simulink model "AHRS_voter_Harness3"  (R2018b)
settings: Solver=FixedStepDiscrete  StartTime=0.0  StopTime=10.0  FixedStep=0.01  RelTol=1e-3  EnableMultiTasking=on
Description:
  | Harness for testing 3 valid AHRS
settings Model: Creator=bpotter  LastModifiedBy=bpotter
settings DataIOCC: LimitDataPoints=on  SaveOutput=off  DSMLogging=off  InspectSignalLogs=on  SaveTime=off
settings OptimizationCC: BlockReduction=off  DefaultParameterBehavior=Inlined  InitFltsAndDblsToZero=on  EfficientFloat2IntCast=on  EfficientMapNaN2IntZero=off  LifeSpan=inf  MaxStackSize=inf
settings DebuggingCC: SignalInfNanChecking=error  SignalRangeChecking=error  ReadBeforeWriteMsg=EnableAllAsError  WriteAfterWriteMsg=EnableAllAsError  WriteAfterReadMsg=EnableAllAsError  AlgebraicLoopMsg=error  ArtificialAlgebraicLoopMsg=error  SaveWithDisabledLinksMsg=error  SaveWithParameterizedLinksMsg=error  BlockPriorityViolationMsg=error  SolverPrmCheckMsg=error  InheritedTsInSrcMsg=error  SigSpecEnsureSampleTimeMsg=error  CheckMatrixSingularityMsg=error  IntegerOverflowMsg=error  ParameterUnderflowMsg=error  ParameterPrecisionLossMsg=error  ParameterTunabilityLossMsg=error  UnderSpecifiedDataTypeMsg=error  UnnecessaryDatatypeConvMsg=warning  VectorMatrixConversionMsg=error  SignalLabelMismatchMsg=error  UnconnectedInputMsg=error  UnconnectedOutputMsg=error  UnconnectedLineMsg=error  SFcnCompatibilityMsg=error  BusObjectLabelMismatch=error  RootOutportRequireBusObject=error  AssertControl=DisableAll  AllowSymbolicDim=off  ModelReferenceIOMsg=error  ModelReferenceIOMismatchMessage=error  UnknownTsInhSupMsg=error  ModelReferenceDataLoggingMessage=error  StateNameClashWarn=warning  StrictBusMsg=ErrorOnBusTreatedAsVector  NonBusSignalsTreatedAsBus=error  SFInvalidInputDataAccessInChartInitDiag=error  SFTransitionOutsideNaturalParentDiag=error  SFUnreachableExecutionPathDiag=error  SFUndirectedBroadcastEventsDiag=error  SFTransitionActionBeforeConditionDiag=error  IntegerSaturationMsg=error
settings HardwareCC: ProdBitPerPointer=32  ProdBitPerSizeT=32  ProdBitPerPtrDiffT=32  ProdLargestAtomicFloat=None  ProdEndianess=Unspecified  ProdWordSize=32  ProdHWDeviceType=32-bit Generic  TargetIntDivRoundTo=Zero
settings ModelReferenceCC: PropagateSignalLabelsOutOfModel=off
settings SFSimCC: SimUseLocalCustomCode=off  MATLABDynamicMemAlloc=off
settings RTWCC: SystemTargetFile=ert.tlc  TemplateMakefile=ert_default_tmf  GenerateReport=on  RTWUseLocalCustomCode=off  IncludeHyperlinkInReport=on  LaunchReport=on  PortableWordSizes=on  GenerateTraceInfo=on  GenerateTraceReport=on  GenerateTraceReportSl=on  GenerateTraceReportSf=on  GenerateTraceReportEml=on
settings CodeAppCC: ForceParamTrailComments=on  IgnoreCustomStorageClasses=off  MangleLength=4  StateflowObjectComments=on  ReqsInCode=on
settings ERTTargetCC: UtilityFuncGeneration=Shared location  MultiwordLength=2048  GenerateSampleERTMain=on  IncludeMdlTerminateFcn=off  GeneratePreprocessorConditionals=Disable all  SuppressErrorStatus=on  SupportAbsoluteTime=off  SupportNonFinite=off  ParenthesesLevel=Maximum  GenerateSharedConstants=off  ERTCustomFileTemplate=example_file_process.tlc  PreserveExpressionOrder=on  PreserveIfCondition=on  ConvertIfToSwitch=off  SuppressUnreachableDefaultCases=off
settings ConfigComp: CovEnable=on  CovScope=ReferencedModels  CovIncludeTopModel=off  CovMetricSettings=dcmtrzoibe  CovHTMLOptions=-sRT=1 -sVT=0 -aTS=0 -bRG=1 -bTC=1 -hTR=1 -nFC=0 -nFD=1 -scm=1 -bcm=1 -xEv=0 -xEM=0  CovHtmlReporting=on  CovSaveCumulativeToWorkspaceVar=on  CovCumulativeVarName=AHRScovCumData  CovCumulativeReport=on  CovModelRefEnable=all  CovExternalEMLEnable=off  CovSFcnEnable=off  PSVerificationMode=BugFinder  PSResultDir=Bugfinder_results_$ModelName$  PSAutoStubLUT=off

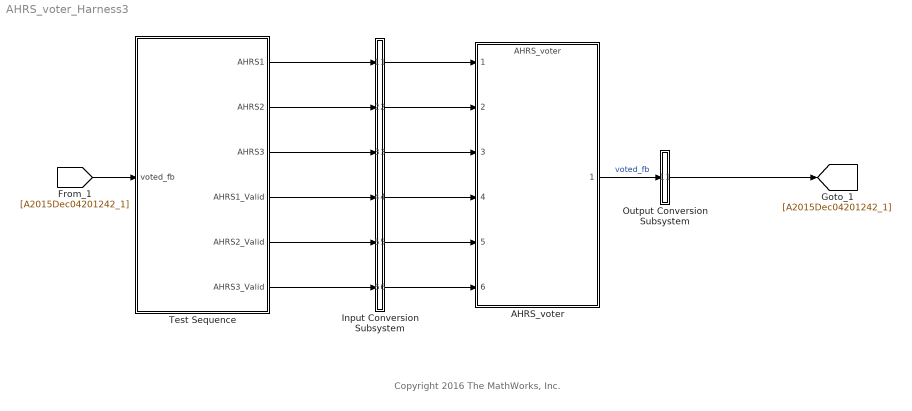
== system AHRS_voter_Harness3 ==
  note: Copyright 2016 The MathWorks, Inc.
  AHRS_voter : ModelReference  ModelNameDialog=AHRS_voter  SimulationMode=Normal  ModelReferenceVersion=1.56
  Input Conversion Subsystem : Subsystem  Tag=__SLT_ICS__
  Output Conversion Subsystem : Subsystem  Tag=__SLT_OCS__
  Test Sequence : Test Sequence  TreatAsAtomicUnit=on
  wires:
  [A2015Dec04201242_1] -> Test Sequence/1(voted_fb)
  Test Sequence/1(AHRS1) -> Input Conversion Subsystem/1(In_1)
  Test Sequence/2(AHRS2) -> Input Conversion Subsystem/2(In_2)
  Test Sequence/3(AHRS3) -> Input Conversion Subsystem/3(In_3)
  Test Sequence/4(AHRS1_Valid) -> Input Conversion Subsystem/4(In_4)
  Test Sequence/5(AHRS2_Valid) -> Input Conversion Subsystem/5(In_5)
  Test Sequence/6(AHRS3_Valid) -> Input Conversion Subsystem/6(In_6)
  Input Conversion Subsystem/1(Out_1) -> AHRS_voter/1
  Input Conversion Subsystem/2(Out_2) -> AHRS_voter/2
  Input Conversion Subsystem/3(Out_3) -> AHRS_voter/3
  Input Conversion Subsystem/4(Out_4) -> AHRS_voter/4
  Input Conversion Subsystem/5(Out_5) -> AHRS_voter/5
  Input Conversion Subsystem/6(Out_6) -> AHRS_voter/6
  AHRS_voter/1 -> Output Conversion Subsystem/1(In_1)  "voted_fb"
  Output Conversion Subsystem/1(Out_1) -> [A2015Dec04201242_1]

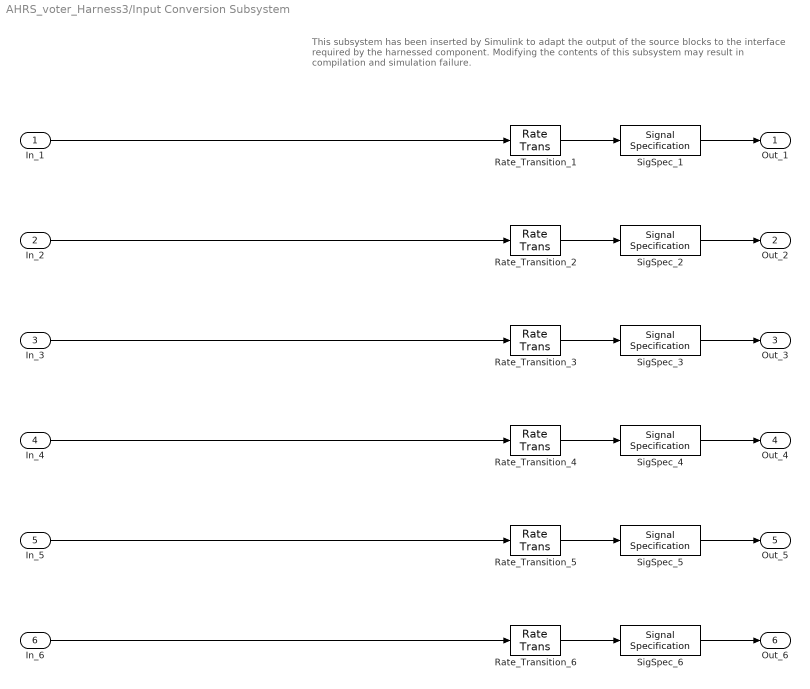
== system AHRS_voter_Harness3/Input Conversion Subsystem ==
  note: This subsystem has been inserted by Simulink to adapt the output of the source blocks to the interface required by the harnessed component.
      |  Modifying the contents of this subsystem may result in compilation and simulation failure.
  In_1 : Inport
  In_2 : Inport  Port=2
  In_3 : Inport  Port=3
  In_4 : Inport  Port=4
  In_5 : Inport  Port=5
  In_6 : Inport  Port=6
  Rate_Transition_{1..6} (6 alike) : RateTransition  OutPortSampleTime=0.01
  SigSpec_1 : SignalSpecification  OutDataTypeStr=double  Dimensions=[5]  SampleTime=0.01
  SigSpec_2 : SignalSpecification  OutDataTypeStr=double  Dimensions=[5]  SampleTime=0.01
  SigSpec_3 : SignalSpecification  OutDataTypeStr=double  Dimensions=[5]  SampleTime=0.01
  SigSpec_4 : SignalSpecification  OutDataTypeStr=boolean  Dimensions=[1]  SampleTime=0.01
  SigSpec_5 : SignalSpecification  OutDataTypeStr=boolean  Dimensions=[1]  SampleTime=0.01
  SigSpec_6 : SignalSpecification  OutDataTypeStr=boolean  Dimensions=[1]  SampleTime=0.01
  Out_1 : Outport
  Out_2 : Outport  Port=2
  Out_3 : Outport  Port=3
  Out_4 : Outport  Port=4
  Out_5 : Outport  Port=5
  Out_6 : Outport  Port=6
  wires:
  In_1/1 -> Rate_Transition_1/1
  In_2/1 -> Rate_Transition_2/1
  In_3/1 -> Rate_Transition_3/1
  In_4/1 -> Rate_Transition_4/1
  In_5/1 -> Rate_Transition_5/1
  In_6/1 -> Rate_Transition_6/1
  Rate_Transition_1/1 -> SigSpec_1/1
  Rate_Transition_2/1 -> SigSpec_2/1
  Rate_Transition_3/1 -> SigSpec_3/1
  Rate_Transition_4/1 -> SigSpec_4/1
  Rate_Transition_5/1 -> SigSpec_5/1
  Rate_Transition_6/1 -> SigSpec_6/1
  SigSpec_1/1 -> Out_1/1
  SigSpec_2/1 -> Out_2/1
  SigSpec_3/1 -> Out_3/1
  SigSpec_4/1 -> Out_4/1
  SigSpec_5/1 -> Out_5/1
  SigSpec_6/1 -> Out_6/1

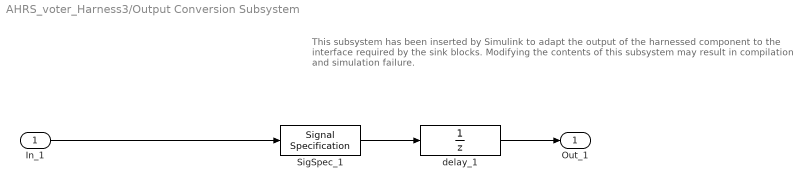
== system AHRS_voter_Harness3/Output Conversion Subsystem ==
  note: This subsystem has been inserted by Simulink to adapt the output of the harnessed component to the interface required by the sink blocks.
      |  Modifying the contents of this subsystem may result in compilation and simulation failure.
  In_1 : Inport
  SigSpec_1 : SignalSpecification  OutDataTypeStr=double  Dimensions=[5]  SampleTime=0.01
  delay_1 : UnitDelay  SampleTime=-1
  Out_1 : Outport
  wires:
  delay_1/1 -> Out_1/1
  SigSpec_1/1 -> delay_1/1
  In_1/1 -> SigSpec_1/1

== stateflow chart AHRS_voter_Harness3/Test Sequence ==
  settings: stateMachineType=SIMPLIFIED_MACHINE
  state step_1
    % Set all data to zero
    AHRS1 = zeros(5, 1);
    AHRS2 = zeros(5, 1);
    AHRS3 = zeros(5, 1);
    % Set all AHRS valid
    AHRS1_Valid = true;
    AHRS2_Valid = true;
    AHRS3_Valid = true;
  state step_2
    % Test that all outputs are set to zero uisng the tolerance
    verify(abs(voted_fb(1))<Tol, 'Zero output condition failed for Parameter1');
    verify(abs(voted_fb(2))<Tol, 'Zero output condition failed for Parameter2');
    verify(abs(voted_fb(3))<Tol, 'Zero output condition failed for Parameter3');
    verify(abs(voted_fb(4))<Tol, 'Zero output condition failed for Parameter4');
    verify(abs(voted_fb(5))<Tol, 'Zero output condition failed for Parameter5');
  state step_3
    % Set data to different values for each AHRS and each element
    AHRS1 = [1; -2; 3; 4; 0;];
    AHRS2 = [-1; 2; -3; -4; -5;];
    AHRS3 = [5; 4; 3; -2; 1;];
  state step_4
    % Test that each element is the mid value, based on the three inputs
    verify((voted_fb(1)-AHRS1(1))<Tol, 'Mid value selection failed for AHRS1 Parameter1');
    verify((voted_fb(2)-AHRS2(2))<Tol, 'Mid value selection failed for AHRS2 Parameter2');
    verify((voted_fb(3)-AHRS3(3))<Tol, 'Mid value selection failed for AHRS3 Parameter3');
    verify((voted_fb(4)-AHRS3(4))<Tol, 'Mid value selection failed for AHRS3 Parameter4');
    verify((voted_fb(5)-AHRS1(5))<Tol, 'Mid value selection failed for AHRS1 Parameter5');
  state step_5
    % Set data to different vlaues at or near full positive range for each AHRS and each element
    AHRS1 = [180; 179; 180; 178; 178;];
    AHRS2 = [179; 180; 179; 179; 180;];
    AHRS3 = [178; 178; 178; 180; 179;];
  state step_6
    % Test that each element is the mid value, based on the three inputs
    verify((voted_fb(1)-AHRS2(1))<Tol, 'Mid value selection failed for AHRS2 Parameter1');
    verify((voted_fb(2)-AHRS1(2))<Tol, 'Mid value selection failed for AHRS1 Parameter2');
    verify((voted_fb(3)-AHRS2(3))<Tol, 'Mid value selection failed for AHRS2 Parameter3');
    verify((voted_fb(4)-AHRS2(4))<Tol, 'Mid value selection failed for AHRS2 Parameter4');
    verify((voted_fb(5)-AHRS3(5))<Tol, 'Mid value selection failed for AHRS3 Parameter5');
  state step_7
    % Set data to different vlaues at or near full negative range for each AHRS and each element
    AHRS1 = [-180; -178; -179; -179; -180;];
    AHRS2 = [-178; -180; -180; -178; -179;];
    AHRS3 = [-179; -179; -178; -180; -178;];
  state step_8
    % Test that each element is the mid value, based on the three inputs
    verify((voted_fb(1)-AHRS3(1))<Tol, 'Mid value selection failed for AHRS3 Parameter1');
    verify((voted_fb(2)-AHRS3(2))<Tol, 'Mid value selection failed for AHRS3 Parameter2');
    verify((voted_fb(3)-AHRS1(3))<Tol, 'Mid value selection failed for AHRS1 Parameter3');
    verify((voted_fb(4)-AHRS1(4))<Tol, 'Mid value selection failed for AHRS1 Parameter4');
    verify((voted_fb(5)-AHRS2(5))<Tol, 'Mid value selection failed for AHRS2 Parameter5');
  (default) -> step_1
  step_1 -> step_2 : [after(1, sec)]
  step_2 -> step_3
  step_3 -> step_4 : [after(1, sec)]
  step_4 -> step_5
  step_5 -> step_6 : [after(1, sec)]
  step_6 -> step_7
  step_7 -> step_8 : [after(1, sec)]
  data: voted_fb input double size=[5]; AHRS1 output double size=[5]; AHRS2 output double size=[5]; AHRS3 output double size=[5]; AHRS1_Valid output boolean size=[1]; AHRS2_Valid output boolean size=[1]; AHRS3_Valid output boolean size=[1]; Tol constant double =1e-7
